simulink model "SimulinkEnv_o"  (R2024a)
settings: Solver=FixedStepAuto  StartTime=0.0  StopTime=8  FixedStep=0.01  RelTol=1e-3
InitFcn:
  | map = load(fullfile('.', '/Resources/map.mat'));
  | 
  | R_uc2rc = map.worldObjectStruct.transforms.rotm_simcam2gencam;
  | 
  | R_uw2rw = map.worldObjectStruct.transforms.rotm_sim2world;
model workspace (MAT data in the model file):
  SL_ROS_VariableLengthArrays_MaxSizes.CommonInfo.ArrayTruncateAction = 'EmitWarning'
  SL_ROS_VariableLengthArrays_MaxSizes.MsgTypeMap = containers.Map
  SL_ROS_VariableLengthArrays_MaxSizes.MsgTypeMap.serialization.keys = {'sensor_msgs/Image'}
  SL_ROS_VariableLengthArrays_MaxSizes.MsgTypeMap.serialization.values{1}(1).PropertyName = 'data'
  SL_ROS_VariableLengthArrays_MaxSizes.MsgTypeMap.serialization.values{1}(1).DataType = 'uint8'
  SL_ROS_VariableLengthArrays_MaxSizes.MsgTypeMap.serialization.values{1}(1).MaxLength = 2764800
  SL_ROS_VariableLengthArrays_MaxSizes.MsgTypeMap.serialization.values{1}(2).PropertyName = 'encoding'
  SL_ROS_VariableLengthArrays_MaxSizes.MsgTypeMap.serialization.values{1}(2).DataType = 'uint8'
  SL_ROS_VariableLengthArrays_MaxSizes.MsgTypeMap.serialization.values{1}(2).MaxLength = 128
  SL_ROS_VariableLengthArrays_MaxSizes.MsgTypeMap.serialization.uniformity = 0
  SL_ROS_VariableLengthArrays_MaxSizes.MsgTypeMap.serialization.keyType = 'char'
  SL_ROS_VariableLengthArrays_MaxSizes.MsgTypeMap.serialization.valueType = 'any'
undefined symbols (not defined in the file or in its folder): Sim3dSensor
libraries: sim3dlib x5, simulink x4, robotcorelib x2, shared6dof x1, shareduavrstlib x1, sim3dcameralib x1, uavsim3dlib x1, dspvision x1, visionsinks x1
settings Model: PauseTimes=0.5  Creator=dylanfanner  LastModifiedBy=alyss
settings OptimizationCC: EnhancedBackFolding=on  PassReuseOutputArgsAs=Individual arguments  ZeroExternalMemoryAtStartup=off  ZeroInternalMemoryAtStartup=off  MaxStackSize=64  OptimizeBlockOrder=speed  DifferentSizesBufferReuse=on  OptimizationCustomize=off  EfficientTunableParamExpr=on
settings DebuggingCC: ParameterTunabilityLossMsg=error
settings HardwareCC: ProdBitPerLong=64  ProdHWDeviceType=Intel->x86-64 (Linux 64)
settings SFSimCC: MATLABDynamicMemAlloc=off
settings RTWCC: Description=Embedded Coder  SystemTargetFile=ert.tlc  HardwareBoard=Robot Operating System 2 (ROS 2)  TLCOptions="-aInlineSetEventsForThisBaseRateFcn=TLC_FALSE -aSuppressMultiTaskScheduler=TLC_FALSE  -aRateBasedStepFcn=0"  TemplateMakefile=ert_default_tmf  Toolchain=Colcon Tools  TargetLang=C++
settings CodeAppCC: ForceParamTrailComments=on  IgnoreCustomStorageClasses=off  OperatorAnnotations=on  SimulinkDataObjDesc=on  SFDataObjDesc=on  InsertBlockDesc=on
settings ERTTargetCC: CodeInterfacePackaging=C++ class  RootIOFormat=Structure reference

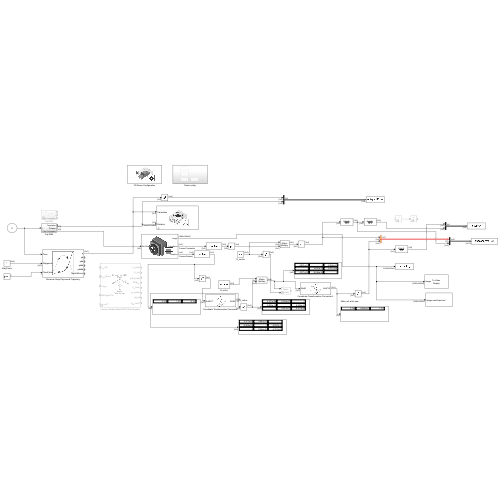
[thumbnail: Simulink's stored preview of the top-level diagram]
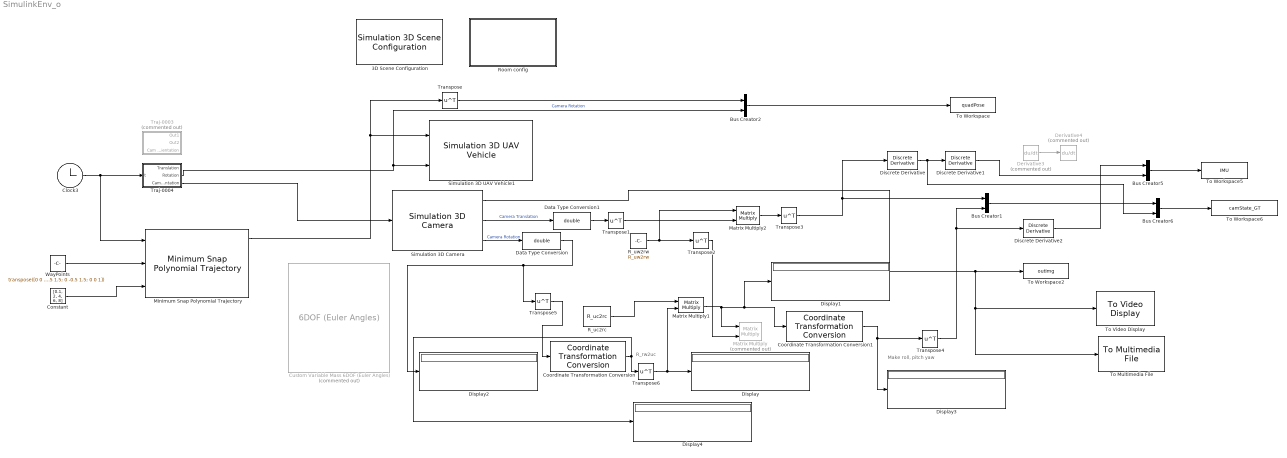
== system SimulinkEnv_o ==
  note: R_rw2uc
  note: Make roll, pitch yaw
  3D Scene Configuration : sim3dlib/Simulation 3D Scene Configuration  Priority=0  ProjectFormat=Default Scenes  SceneDesc=Empty scene  ProjectName=C:\Programs\MATLAB\R2024a\toolbox\shared\sim3d_projects\automotive_project_windows\UE\WindowsNoEditor\VehicleSimulation.exe  ScenePath=/Game/Maps/HwStrght  EnableOpenDRIVE=off  vehTagList={'Custom';'GenericQuad1';'Scene Origin';'Sim3dActor1';'Sim3dActor2';'Sim3dActor3';'Sim3dActor4'}  vehTag=Scene Origin  FreeCameraInitialTranslation=[0, 0, 0]  FreeCameraDefaultInitialTranslation=[-6, 0, 2]  FreeCameraInitialRotation=[0, 0, 0]  FreeCameraDefaultInitialRotation=[0, -15, 0]  OpVisEn=off  Ts=.01  EnableWindow=on  EnableRemoteAccess=off  EnableWeather=off  SunAzimuth=90  SunAltitude=40.0  EnableGeospatialSun=off  Latitude=0  Longitude=0  Date=2023-01-01  Time=10:30:00  GeoTimeZone=-5.0  SunDaylightSaving=off  wind=1  clouds=10  EnableVolumetricClouds=off  CloudCoverage=0  CloudAltitude=6  fog=0  rain=0  RaindropsEffect=off  SnowDensity=0.0  EnableGeospatial=off  UseTrueOrigin=off  OriginHeight=200  OriginLatitude=40.744652  OriginLongitude=-73.988864  MapStyle=Aerial  AdditionalAssetIDs=[]  UseAdvancedSunSky=off  SolarTime=11  TimeZone=-5  Day=21  Month=9  Year=2022  UseDaylightSavingTime=on  DSTStartDay=10  DSTStartMonth=3  DSTEndDay=3  DSTEndMonth=11  DSTSwitchHour=2  sensorTag=MainCamera1  sensorId=1  sensorName=MainCamera1  mountLoc=Origin  offsetFlag=off  tmountOffset=[0, 0, 0]  rmountOffset=[0, 0, 0]  HorizontalResolution=1280  VerticalResolution=720  HorizontalFOV=60  mountPoint=[0 0 0]  mountOrientation=[0 0 0]  aMode=5  ID=1  GeoTrigger=Inactive
      settings: LibrarySourceBlock=sl3dlib/Simulation 3D/Environment/Simulation 3D Scene Configuration
  Bus Creator1 : BusCreator  Inputs=3
  Bus Creator2 : BusCreator  Inputs=2
  Bus Creator5 : BusCreator  Inputs=2
  Bus Creator6 : BusCreator  Inputs=2
  Clock3 : Clock
  Constant : Constant  Value=[0.1, 2, 4, 6, 8]
  Coordinate Transformation Conversion : robotcorelib/Coordinate Transformation Conversion  InputRepresentation=Euler Angles  InputEulerSequence=XYZ  ShowTrVecInputPort=on  OutputRepresentation=Rotation Matrix  OutputEulerSequence=ZYX  ShowTrVecOutputPort=on  SimulateUsing=Interpreted execution
      settings: LibrarySourceBlock=uavutilslib/Coordinate Transformation Conversion
  Coordinate Transformation Conversion1 : robotcorelib/Coordinate Transformation Conversion  InputRepresentation=Rotation Matrix  InputEulerSequence=XYZ  ShowTrVecInputPort=on  OutputRepresentation=Euler Angles  OutputEulerSequence=XYZ  ShowTrVecOutputPort=on  SimulateUsing=Interpreted execution
      settings: LibrarySourceBlock=uavutilslib/Coordinate Transformation Conversion
  Custom Variable Mass 6DOF (Euler Angles) : shared6dof/6DOF (Euler Angles)  Commented=on  units=Metric (MKS)  mtype=Custom Variable  rep=Euler Angles  xme_0=[0 0 0]  Vm_0=[0 0 0]  eul_0=[0 0 0]  pm_0=[0 0 0]  mass_0=1.0  mass_e=0.5  mass_f=2.0  inertia=eye(3)  inertia_e=eye(3)  inertia_f=2*eye(3)  k_quat=1.0  vre_flag=off  abi_flag=off  aMode=0  xme_statename=''  Vm_statename=''  eul_statename=''  quat_statename=''  pm_statename=''  mass_statename=''
      settings: LibrarySourceBlock=aerolib6dof2/Custom Variable Mass 6DOF (Euler Angles)
  Data Type Conversion : DataTypeConversion  OutDataTypeStr=double  RndMeth=Nearest  SaturateOnIntegerOverflow=off
  Data Type Conversion1 : DataTypeConversion  OutDataTypeStr=double  RndMeth=Nearest  SaturateOnIntegerOverflow=off
  Derivative3 : Derivative  Commented=on
  Derivative4 : Derivative  Commented=on
  Discrete Derivative : simulink/Discrete/Discrete Derivative  gainval=1.0  ICPrevScaledInput=0.0  OutMin=[]  OutMax=[]  OutDataType=fixdt(1, 16)  OutScaling=2^-10  DoSatur=off
  Discrete Derivative1 : simulink/Discrete/Discrete Derivative  gainval=1.0  ICPrevScaledInput=0.0  OutMin=[]  OutMax=[]  OutDataType=fixdt(1, 16)  OutScaling=2^-10  DoSatur=off
  Discrete Derivative2 : simulink/Discrete/Discrete Derivative  gainval=1.0  ICPrevScaledInput=0.0  OutMin=[]  OutMax=[]  OutDataType=fixdt(1, 16)  OutScaling=2^-10  DoSatur=off
  Display{,1..4} (5 alike) : Display
  Matrix Multiply : Product  Commented=on  Multiplication=Matrix(*)
  Matrix Multiply1 : Product  Multiplication=Matrix(*)
  Matrix Multiply2 : Product  Multiplication=Matrix(*)
  Minimum Snap Polynomial Trajectory : shareduavrstlib/Minimum Snap Polynomial Trajectory  ShowBCInputPort=off  ShowPolynomialCoefs=off  ShowStatusOutputPort=off  TimeAllocation=off  TimeWeight=100  MinSegmentTime=0.1  MaxSegmentTime=1  MaxIteration=1500  MaxTime=10  SimulateUsing=Interpreted execution
      settings: LibrarySourceBlock=uavalgslib/Minimum Snap Polynomial Trajectory
  R_uc2rc : Constant  Value=R_uc2rc
  R_uw2rw : Constant  Value=R_uw2rw
  Room config : Subsystem
  Simulation 3D Camera : sim3dcameralib/Simulation 3D Camera  Priority=1  sensorTag=Sim3dSensor�  sensorId=2  sensorName=Sim3dSensor�  vehTagList={'GenericQuad1';'Scene Origin';'Sim3dActor1';'Sim3dActor2';'Sim3dActor3';'Sim3dActor4'}  vehTag=GenericQuad1  mountLoc=Origin  offsetFlag=on  tmountOffset=[0, 0, 0]  extTmount=off  rmountOffset=[0, 0, 0]  extRmount=on  FocalLength=[1107, 1107]  OpticalCenter=[640*1.5, 360*1.5]  ImageSize=[720*1.5, 1280*1.5]  RadialDistortion=[0, 0]  TangentialDistortion=[0, 0]  SensorSkew=0  DepthOutportEnabled=off  SemanticOutportEnabled=off  TransformOutportEnabled=on  SampleTime=0.05  mountPoint=[0 0 0]  mountOrientation=[0 0 0]  aMode=6  ID=2
      settings: LibrarySourceBlock=robotsim3dlib/Simulation 3D Camera
  Simulation 3D UAV Vehicle1 : uavsim3dlib/Simulation 3D UAV Vehicle  Priority=-1  Mesh=Quadrotor  MeshPath=/MathWorksUAVContent/UAVs/HexaRotorUAV/HexaRotor.HexaRotor  Color=Black  ActorName=GenericQuad1  UseGlobalFrame=off  InitialTranslation=[0 0 0]  InitialRotation=[0 0 0]  InitialTranslationGlobal=[0 0 0]  InitialGeoOrigin=[0 0 0]  InitialRotationGlobal=[0 0 0]  SampleTime=-1  ActorType=SimulinkVehicle  ID=C  aMode=4  ActorTag=GenericQuad1
  To Multimedia File : dspvision/To Multimedia File  outputFilename=camOutput.avi  streamSelection=Video only  videoCompressor=None (uncompressed)  audioCompressor=None (uncompressed)  imagePorts=One multidimensional signal  fileType=AVI  audioDatatype=Determine from input data type  fourcc=RGB  audioBitRate=128  audioQuality=75  videoQuality=75  mj2000CompFactor=10
      settings: LibrarySourceBlock=visionsinks/To Multimedia File
  To Video Display : visionsinks/To Video Display  windowSizeMode=Normal  openAtMdlStart=on  fullScreen=off  videoWindowX=0  videoWindowY=23  saveWindowSize=off  videoWindowWidth=1366  videoWindowHeight=745  inputColorFormat=RGB  inputType=Obsolete  imagePorts=One multidimensional signal  OutputDevice=On-screen video monitor  dataOrg=Column-major  isWindowOpen=off
  To Workspace : ToWorkspace  VariableName=quadPose  SaveFormat=Structure With Time  SampleTime=0.01
  To Workspace2 : ToWorkspace  VariableName=outImg  SaveFormat=Structure With Time  SampleTime=0.1
  To Workspace5 : ToWorkspace  VariableName=IMU  SaveFormat=Structure With Time  SampleTime=0.05
  To Workspace6 : ToWorkspace  VariableName=camState_GT  SaveFormat=Structure With Time  SampleTime=0.05
  Traj-0003 : Subsystem  Commented=on
  Traj-0004 : Subsystem
  Transpose{,1..6} (7 alike) : Math  Operator=transpose
  WayPoints : Constant  Value=transpose([0 0 0; 0 0 1; 0 0.5 1.5; 0 -0.5 1.5; 0 0 1])
  wires:
  Simulation 3D Camera/1 -> To Workspace2/1, To Video Display/1, To Multimedia File/1
  Traj-0004/2(Rotation) -> Bus Creator2/2, Simulation 3D UAV Vehicle1/2  "Camera Rotation"
  Bus Creator1/1 -> Bus Creator6/1
  Minimum Snap Polynomial Trajectory/1 -> Transpose/1, Simulation 3D UAV Vehicle1/1
  Traj-0004/3(Cam Orientation) -> Simulation 3D Camera/1
  Bus Creator2/1 -> To Workspace/1
  Clock3/1 -> Minimum Snap Polynomial Trajectory/1, Traj-0004/1(t)
  WayPoints/1 -> Minimum Snap Polynomial Trajectory/2
  Constant/1 -> Minimum Snap Polynomial Trajectory/3
  Transpose/1 -> Bus Creator2/1
  Bus Creator6/1 -> To Workspace6/1
  Derivative3/1 -> Derivative4/1
  Bus Creator5/1 -> To Workspace5/1
  Simulation 3D Camera/3 -> Data Type Conversion/1  "Camera Rotation"
  Simulation 3D Camera/2 -> Data Type Conversion1/1  "Camera Translation"
  R_uw2rw/1 -> Transpose2/1, Matrix Multiply2/1
  Data Type Conversion1/1 -> Transpose1/1
  Transpose1/1 -> Matrix Multiply2/2
  Discrete Derivative1/1 -> Bus Creator5/2
  Discrete Derivative2/1 -> Bus Creator5/1
  Discrete Derivative/1 -> Bus Creator6/2, Discrete Derivative1/1
  Matrix Multiply1/1 -> Display1/1, Coordinate Transformation Conversion1/1, Matrix Multiply/1
  Transpose2/1 -> Matrix Multiply/2
  Matrix Multiply2/1 -> Transpose3/1
  Transpose3/1 -> Bus Creator1/1, Discrete Derivative/1
  Data Type Conversion/1 -> Transpose5/1, Display2/1
  Coordinate Transformation Conversion1/1 -> Display3/1, Transpose4/1
  Transpose4/1 -> Discrete Derivative2/1, Bus Creator1/3
  R_uc2rc/1 -> Matrix Multiply1/1
  Transpose5/1 -> Coordinate Transformation Conversion/1
  Coordinate Transformation Conversion/1 -> Transpose6/1, Display4/1
  Transpose6/1 -> Matrix Multiply1/2, Display/1

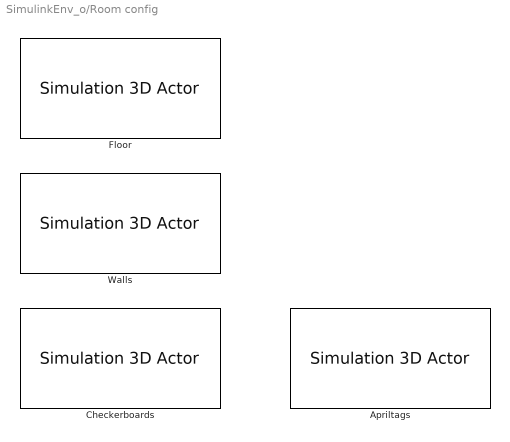
== system SimulinkEnv_o/Room config ==
  Apriltags : sim3dlib/Simulation 3D Actor  Priority=1  ActorName=Sim3dActor1  ParentName=Scene Origin  Operation=Create at setup  InitScriptText=|  SampleTime=-1  Translation=single([0 0 0])  Rotation=single([0 0 0])  Scale=single([1 1 1])  aMode=5  ActorTag=Sim3dActor1  ActorType=Sim3dActor  ID=1
      | % Reserved keywords:
      | % - Actor : handle to this actor object
      | % - World : handle to the world object
      | 
      | % Examples:
      | 
      | % Create a primitive geometry (optional)
      | % Actor.createShape('box', [1 1 1]);
      | 
      | % Initialize values (optional)
      | % Actor.Scale = 1;
      | % Actor.Color = [1 0 0];
  Checkerboards : sim3dlib/Simulation 3D Actor  Priority=1  ActorName=Sim3dActor2  ParentName=Scene Origin  Operation=Create at setup  InitScriptText=|  SampleTime=-1  Translation=single([0 0 0])  Rotation=single([0 0 0])  Scale=single([1 1 1])  aMode=5  ActorTag=Sim3dActor2  ActorType=Sim3dActor  ID=2
      | % Reserved keywords:
      | % - Actor : handle to this actor object
      | % - World : handle to the world object
      | 
      | % Examples:
      | 
      | % Create a primitive geometry (optional)
      | % Actor.createShape('box', [1 1 1]);
      | 
      | % Initialize values (optional)
      | % Actor.Scale = 1;
      | % Actor.Color = [1 0 0];
  Floor : sim3dlib/Simulation 3D Actor  Priority=1  ActorName=Sim3dActor3  ParentName=Scene Origin  Operation=Create at setup  InitScriptText=|  SampleTime=-1  Translation=single([0 0 0])  Rotation=single([0 0 0])  Scale=single([1 1 1])  aMode=5  ActorTag=Sim3dActor3  ActorType=Sim3dActor  ID=3
      | % Reserved keywords:
      | % - Actor : handle to this actor object
      | % - World : handle to the world object
      | 
      | % Examples:
      | 
      | % Create a primitive geometry (optional)
      | % Actor.createShape('box', [1 1 1]);
      | 
      | % Initialize values (optional)
      | % Actor.Scale = 1;
      | % Actor.Color = [1 0 0];
  Walls : sim3dlib/Simulation 3D Actor  Priority=1  ActorName=Sim3dActor4  ParentName=Scene Origin  Operation=Create at setup  InitScriptText=|  SampleTime=-1  Translation=single([0 0 0])  Rotation=single([0 0 0])  Scale=single([1 1 1])  aMode=5  ActorTag=Sim3dActor4  ActorType=Sim3dActor  ID=4
      | % Reserved keywords:
      | % - Actor : handle to this actor object
      | % - World : handle to the world object
      | 
      | % Examples:
      | 
      | % Create a primitive geometry (optional)
      | % Actor.createShape('box', [1 1 1]);
      | 
      | % Initialize values (optional)
      | % Actor.Scale = 1;
      | % Actor.Color = [1 0 0];

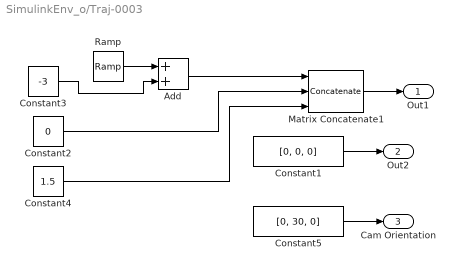
== system SimulinkEnv_o/Traj-0003 ==
  Add : Sum
  Constant1 : Constant  Value=[0, 0, 0]  VectorParams1D=off
  Constant2 : Constant  Value=0
  Constant3 : Constant  Value=-3
  Constant4 : Constant  Value=1.5
  Constant5 : Constant  Value=[0, 30, 0]  VectorParams1D=off
  Matrix Concatenate1 : Concatenate  NumInputs=3  Mode=Multidimensional array  ConcatenateDimension=2
  Ramp : simulink/Sources/Ramp  slope=0.5  start=0.2  InitialOutput=0
  Out1 : Outport
  Out2 : Outport  Port=2
  Cam Orientation : Outport  Port=3
  wires:
  Constant3/1 -> Add/2
  Ramp/1 -> Add/1
  Matrix Concatenate1/1 -> Out1/1
  Add/1 -> Matrix Concatenate1/1
  Constant1/1 -> Out2/1
  Constant2/1 -> Matrix Concatenate1/2
  Constant4/1 -> Matrix Concatenate1/3
  Constant5/1 -> Cam Orientation/1

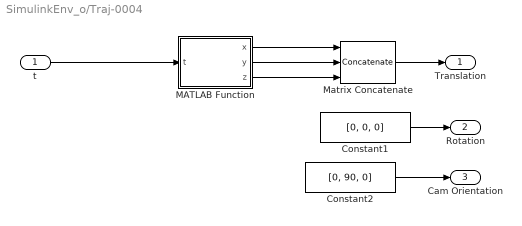
== system SimulinkEnv_o/Traj-0004 ==
  t : Inport
  Constant1 : Constant  Value=[0, 0, 0]  VectorParams1D=off
  Constant2 : Constant  Value=[0, 90, 0]  VectorParams1D=off
  MATLAB Function : MATLAB Function  TreatAsAtomicUnit=on
  Matrix Concatenate : Concatenate  NumInputs=3  Mode=Multidimensional array  ConcatenateDimension=2
  Translation : Outport
  Rotation : Outport  Port=2
  Cam Orientation : Outport  Port=3
  wires:
  t/1 -> MATLAB Function/1(t)
  MATLAB Function/2(y) -> Matrix Concatenate/2
  MATLAB Function/3(z) -> Matrix Concatenate/3
  Matrix Concatenate/1 -> Translation/1
  MATLAB Function/1(x) -> Matrix Concatenate/1
  Constant1/1 -> Rotation/1
  Constant2/1 -> Cam Orientation/1

== matlab function SimulinkEnv_o/Traj-0004/MATLAB Function ==
  data: x output; y output; z output; t input
function [x, y, z] = fcn(t)

    
    %t = get_param(gcs, 'SimulationTime');

    x = 0;
    y = 0;
    z = (1.5/2)*t;
    
    if t>=2
        x =0;
        y=(0.2/2)*t;
        z=1.5;
    end
    
    if t>=4
        x =0;
        y=0.1*(-t+6);
        z=(0.3/2)*t+0.9;
    end
    
    if t>=6
        x =0;
        y=0.1*(-t+6);
        z=1.8;
    end
    
    if t>=8
        x=0;
        y=0.1*(t-10);
        z=(-0.15*t)+3;
    end

end
